simulink model "c6416dskDIPswitch"  (Simulink 6.0)
settings: Solver=FixedStepDiscrete  StartTime=0.0  StopTime=inf  RelTol=1e-3
undefined symbols (not defined in the file): bit
libraries: dspsigops x5, c6416dsklib x4, c6000tgtpreflib x1
settings Model: Creator=zgalijas  LastModifiedBy=thartley  RTWExpressionDepthLimit=1  ProdHWDeviceType=TI C6000
settings DataIOCC: LimitDataPoints=off  SaveOutput=off  SaveTime=off  SignalLoggingName=sigsOut
settings OptimizationCC: InlineParams=on  InlineInvariantSignals=off  EnforceIntegerDowncast=off
settings DebuggingCC: CheckExecutionContextPreStartOutputMsg=on  CheckExecutionContextRuntimeOutputMsg=on  SolverPrmCheckMsg=none
settings HardwareCC: ProdBitPerLong=40  ProdEndianess=LittleEndian  ProdHWDeviceType=TI C6000
settings ModelReferenceCC: UpdateModelReferenceTargets=IfOutOfDate
settings RTWCC: SystemTargetFile=ti_c6000.tlc  TemplateMakefile=ti_c6000.tmf  ProcessScript=ti_c6000_make_rtw_hook
settings CodeAppCC: PrefixModelToSubsysFcnNames=off
settings STFCustomTargetCC: TargetFcnLib=ansi_tfl_tmw.mat  MatFileLogging=on  LifeSpan=inf  SystemTargetFile=ti_c6000.tlc  ActivateCallback=c6000_callback('ActivateCallback',hSrc,hDlg);
settings GRTTargetCC: ModelReferenceCompliant=off  LifeSpan=inf
settings CustomProperty: DataType=RTWOptions_EnumType_S__A_matlab_toolbox_rtw_targets_tic6000_tic6000_ti_c6000_BoardType  Value=C6416DSK
settings EnumStrPairs: String=C6416DSK
settings SFSimCC: SFSimApplyToAllLibs=on  SFSimBuildMode=Incremental

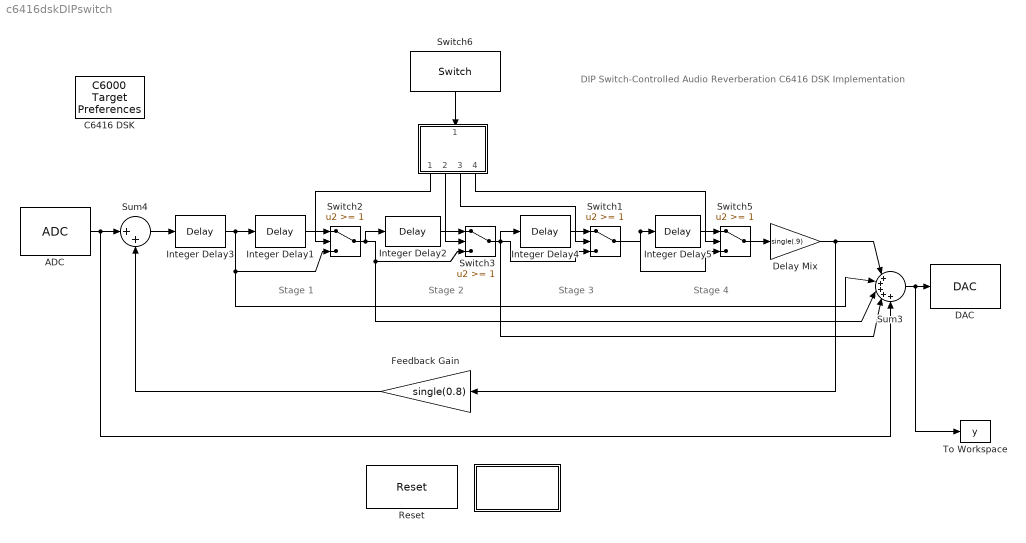
== system c6416dskDIPswitch ==
  note: DIP Switch-Controlled Audio Reverberation
      | C6416 DSK Implementation
  note: Stage 1
  note: Stage 2
  note: Stage 3
  note: Stage 4
  " " : Subsystem
      mask Display: disp('Info')
  "  " : Subsystem  Orientation=down
  ADC : c6416dsklib/ADC  ADCsource=Mic In  MicGain=off  Stereo=on  SampleRate=32 kHz  CodecDataFormat=32-bit  OutputDataType=Single  Scaling=Normalize  SourceGain=0.0  FrameSize=64
  C6416 DSK : c6000tgtpreflib/C6000 Target Preferences
  DAC : c6416dsklib/DAC  CodecDataFormat=32-bit  Scaling=Normalize  DacAtten=0.0  OverflowMode=Saturate
  Delay Mix : Gain  Gain=single(.9)  SaturateOnIntegerOverflow=on
  Feedback Gain : Gain  Orientation=left  Gain=single(0.8)  SaturateOnIntegerOverflow=on
  Integer Delay1 : dspsigops/Delay  dly_unit=Samples  delay=641  ic_detail=off  dif_ic_for_ch=off  dif_ic_for_dly=off  ic=0  reset_popup=None
  Integer Delay2 : dspsigops/Delay  dly_unit=Samples  delay=237  ic_detail=off  dif_ic_for_ch=off  dif_ic_for_dly=off  ic=0  reset_popup=None
  Integer Delay3 : dspsigops/Delay  dly_unit=Samples  delay=300  ic_detail=off  dif_ic_for_ch=off  dif_ic_for_dly=off  ic=0  reset_popup=None
  Integer Delay4 : dspsigops/Delay  dly_unit=Samples  delay=173  ic_detail=off  dif_ic_for_ch=off  dif_ic_for_dly=off  ic=0  reset_popup=None
  Integer Delay5 : dspsigops/Delay  dly_unit=Samples  delay=41  ic_detail=off  dif_ic_for_ch=off  dif_ic_for_dly=off  ic=0  reset_popup=None
  Reset : c6416dsklib/Reset
  Sum3 : Sum  Inputs=|+++++  SaturateOnIntegerOverflow=on  InputSameDT=on
  Sum4 : Sum  Inputs=|++  SaturateOnIntegerOverflow=on  InputSameDT=on
  Switch{1..3,5} (4 alike) : Switch  Threshold=1  ZeroCross=off  InputSameDT=on
  Switch6 : c6416dsklib/Switch  Orientation=down  sw0=on  sw1=on  sw2=on  sw3=on  dType=Boolean  Ts=64/32000
  To Workspace : ToWorkspace  VariableName=y  SampleTime=-1  SaveFormat=Array
  wires:
  Sum3/1 -> DAC/1, To Workspace/1
  ADC/1 -> Sum4/1, Sum3/5
  Feedback Gain/1 -> Sum4/2
  Integer Delay4/1 -> Switch1/1
  Integer Delay1/1 -> Switch2/1
  "  "/1(SW0) -> Switch2/2
  Sum4/1 -> Integer Delay3/1
  Integer Delay3/1 -> Integer Delay1/1, Switch2/3, Sum3/2
  Integer Delay2/1 -> Switch3/1
  "  "/2(SW1) -> Switch3/2
  "  "/3(SW2) -> Switch1/2
  Switch6/1 -> "  "/1("   ")
  Integer Delay5/1 -> Switch5/1
  Switch1/1 -> Switch5/3, Integer Delay5/1
  "  "/4(SW3) -> Switch5/2
  Switch5/1 -> Delay Mix/1
  Switch2/1 -> Integer Delay2/1, Switch3/3, Sum3/3
  Switch3/1 -> Integer Delay4/1, Switch1/3, Sum3/4
  Delay Mix/1 -> Sum3/1, Feedback Gain/1

== system c6416dskDIPswitch/  ==
  note: DIP Switch-Controlled Audio Reverberation
      |
      | This simulation of audio reverberation demonstrates the use of the C6416 DSK DIP Switch block.
      | This block reads the status of user-controlled DIP switches  on the board.
      | Each DIP switch controls a corresponding delay block.

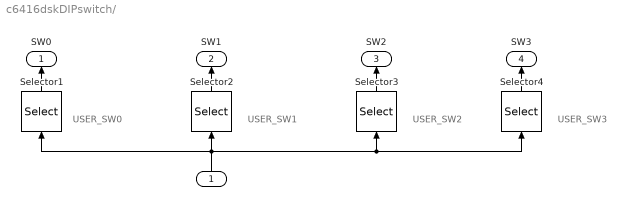
== system c6416dskDIPswitch/   ==
  note: USER_SW0
  note: USER_SW1
  note: USER_SW2
  note: USER_SW3
  "   " : Inport  Orientation=up
  Selector1 : Selector  Orientation=up  InputPortWidth=4
  Selector2 : Selector  Orientation=up  Elements=2  InputPortWidth=4
  Selector3 : Selector  Orientation=up  Elements=3  InputPortWidth=4
  Selector4 : Selector  Orientation=up  Elements=4  InputPortWidth=4
  SW0 : Outport  Orientation=up
  SW1 : Outport  Orientation=up  Port=2
  SW2 : Outport  Orientation=up  Port=3
  SW3 : Outport  Orientation=up  Port=4
  wires:
  "   "/1 -> Selector2/1, Selector1/1, Selector3/1, Selector4/1
  Selector1/1 -> SW0/1
  Selector2/1 -> SW1/1
  Selector3/1 -> SW2/1
  Selector4/1 -> SW3/1
